simulink model "Test_Project_HLC"  (R2018a)
settings: Solver=FixedStepDiscrete  StartTime=0.0  StopTime=inf  FixedStep=1  RelTol=1e-3
undefined symbols (not defined in the file or in its folder): HLC
libraries: simulink x72, powerlib_meascontrol x1
settings Model: DataDictionary=HLC_DD.sldd  Creator=VIJAY BANDEPPA MURGE  LastModifiedBy=VIJAY BANDEPPA MURGE
settings DataIOCC: ReturnWorkspaceOutputs=on
settings SFSimCC: SimUseLocalCustomCode=on
settings RTWCC: RTWUseLocalCustomCode=on

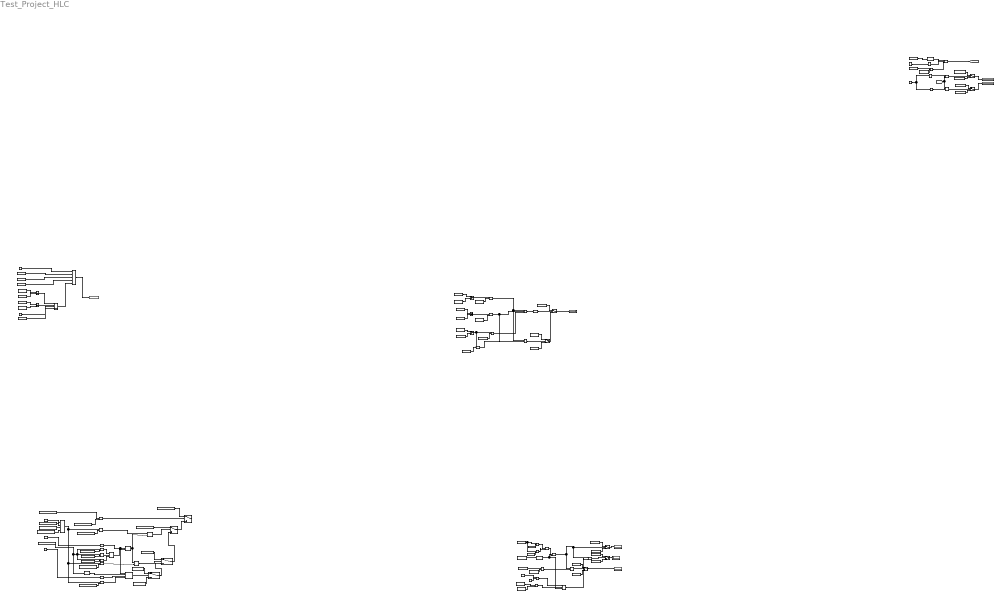
== system Test_Project_HLC ==
  note: Manual
  note: Vijay Murge
      | Road curvature
      | Wheel angle > 7° & Speed > 10km/h & High_Way/Express_Way/ Rural_Road/ Inside_City_Road/ Outside_City_Road
      | Curve_Adaptive_Right_Side_lamp
      |
      | Wheel angle > -7° & Speed > 10km/h & High_Way/Express_Way/ Rural_Road/ Inside_City_Road/ Outside_City_Road
      | Curve_Adaptive_Left_Side_lamp
  note: 4
      | Swapna Nerkar
      | Weather Conditions
      | Fog_Detected/Rain_detected & High_Way/Express_Way/ Rural_Road/Tunnel/Outside_City_Road
      | Fog_Lamp & Parking_Light
      |
      | Fog_Detected/Rain_detected & darkness & High_Way/ Express_Way/ Rural_Road/Tunnel/ Inside_City_Road/Outside_City_Road
      | Low Beam ,fog lamp and parking light
      |
      | Parked Vehicle
      | High_Way/Express_Way/ Rural_Road/Tunnel/Inside_City_Road/ Outside_City_Road & Ignition_On/Ignition_Off & Speed==0
      | Parking_Light
      |
      | Fog_Detected/Rain_detected/Inside_City_Road Fog lamp
  note: 3
      | Snehal Mane
      | Night-time running vehicle
      | Vehicle_Detected at 20m on Left_Side & Darkness & High_Way/Rural_Road/Outside_City_Road
      | Low_Beam -Left_Side_Headlamp
      |
      | Vehicle_Detected at 20m on Left_Side/Right _Side & Darkness & Inside_City_Road
      | Low_Beam
      |
      | Vehicle_Detected at 20m on Right_Side & Darkness & High_Way/Rural_Road/Inside_City_Road/Outside_City_Road
      | Low_Beam -Right_Side_Headlamp
      |
      | Speed > 60km/h & Darkness & No_Vehical_Detected & Inside_City_Road
      | High_Beam
  note: 1
      | Vikrant Gophane
      | Day-time running vehicle
      | Ignition_On/Ignition_Off & Day_Time
      | Headlight_Off
      |
      | Speed > 60km/h & Darkness & High_Way/Express_Way/ Rural_Road/Tunnel/Outside_City_Road
      | High_beam
      |
      | Ignition_On & Day_Time & InSide_City_Road
      | Low_Beam
  note: 2
      | Anupriya Gathekar
      | Day/Night Time but vehicle is in off mode
      | Darkness & Ignition_Off & Vehicle_Locked
      | Low_Beam for 15 Sec.
      |
      | Darkness & Ignition_Off & Vehicle_Unlocked
      | Low_Beam
  note: Auto_Mode
  AND{1,4..5,7..8,12..13} (7 alike) : Logic  IconShape=distinctive  AllPortsSameDT=off  OutDataTypeStr=boolean
  AND10 : Logic  Operator=OR  IconShape=distinctive  AllPortsSameDT=off  OutDataTypeStr=boolean
  AND{2..3,9,11} (4 alike) : Logic  Inputs=3  IconShape=distinctive  AllPortsSameDT=off  OutDataTypeStr=boolean
  AND6 : Logic  Inputs=4  IconShape=distinctive  AllPortsSameDT=off  OutDataTypeStr=boolean
  Angle : Constant  Value=-8
  Compare To Constant1 : simulink/Logic and Bit Operations/Compare To Constant  relop=>=  const=20  OutDataTypeStr=boolean
  Compare To Constant2 : simulink/Logic and Bit Operations/Compare To Constant  relop=>=  const=60  OutDataTypeStr=boolean
  Compare To Constant3 : simulink/Logic and Bit Operations/Compare To Constant  relop=>=  const=7  OutDataTypeStr=boolean
  Compare To Constant4 : simulink/Logic and Bit Operations/Compare To Constant  relop=>=  const=10  OutDataTypeStr=boolean
  Compare To Constant5 : simulink/Logic and Bit Operations/Compare To Constant  relop=<=  const=-7  OutDataTypeStr=boolean
  Constant2 : Constant
  Constant3 : Constant  Value=2
  Constant4 : Constant  Value=0
  Constant5 : Constant  Value=5
  Data Type Conversion : DataTypeConversion
  Data Type Conversion1 : DataTypeConversion
  Data Type Conversion2 : DataTypeConversion  OutDataTypeStr=boolean
  Detection_Distancet : Constant  Value=21
  Display{,1,3..7} (7 alike) : Display
  Enumerated Constant{,15..16,52,54} (5 alike) : simulink/Sources/Enumerated Constant  OutDataTypeStr=Enum: HLC  Value=HLC.Ignition_On  SampleTime=inf
  Enumerated Constant{1,6,17,41} (4 alike) : simulink/Sources/Enumerated Constant  OutDataTypeStr=Enum: HLC  Value=HLC.Day_Time  SampleTime=inf
  Enumerated Constant10 : simulink/Sources/Enumerated Constant  OutDataTypeStr=Enum: HLC  Value=HLC.Ignition_Off  SampleTime=inf
  Enumerated Constant11 : simulink/Sources/Enumerated Constant  OutDataTypeStr=Enum: HLC  Value=HLC.Ignition_Off  SampleTime=inf
  Enumerated Constant12 : simulink/Sources/Enumerated Constant  OutDataTypeStr=Enum: HLC  Value=HLC.Vehicle_locked  SampleTime=inf
  Enumerated Constant13 : simulink/Sources/Enumerated Constant  OutDataTypeStr=Enum: HLC  Value=HLC.Vehicle_Unlocked  SampleTime=inf
  Enumerated Constant{2,4..5,18..19,24,42} (7 alike) : simulink/Sources/Enumerated Constant  OutDataTypeStr=Enum: HLC  Value=HLC.Darkness  SampleTime=inf
  Enumerated Constant20 : simulink/Sources/Enumerated Constant  OutDataTypeStr=Enum: HLC  Value=HLC.Vehicle_locked  SampleTime=inf
  Enumerated Constant{21..22,39,43,65} (5 alike) : simulink/Sources/Enumerated Constant  OutDataTypeStr=Enum: HLC  Value=HLC.Low_Beam  SampleTime=inf
  Enumerated Constant23 : simulink/Sources/Enumerated Constant  OutDataTypeStr=Enum: HLC  Value=HLC.Vehicle_Unlocked  SampleTime=inf
  Enumerated Constant25 : simulink/Sources/Enumerated Constant  OutDataTypeStr=Enum: HLC  Value=HLC.High_Way  SampleTime=inf
  Enumerated Constant26 : simulink/Sources/Enumerated Constant  OutDataTypeStr=Enum: HLC  Value=HLC.Vehicle_Detected_Left  SampleTime=inf
  Enumerated Constant27 : simulink/Sources/Enumerated Constant  OutDataTypeStr=Enum: HLC  Value=HLC.Vehicle_Detected_Right  SampleTime=inf
  Enumerated Constant28 : simulink/Sources/Enumerated Constant  OutDataTypeStr=Enum: HLC  Value=HLC.Rural_Road  SampleTime=inf
  Enumerated Constant29 : simulink/Sources/Enumerated Constant  OutDataTypeStr=Enum: HLC  Value=HLC.Low_Beam_LHS  SampleTime=inf
  Enumerated Constant3 : simulink/Sources/Enumerated Constant  OutDataTypeStr=Enum: HLC  Value=HLC.Ignition_Off  SampleTime=inf
  Enumerated Constant30 : simulink/Sources/Enumerated Constant  OutDataTypeStr=Enum: HLC  Value=HLC.Outside_City_Road  SampleTime=inf
  Enumerated Constant31 : simulink/Sources/Enumerated Constant  OutDataTypeStr=Enum: HLC  Value=HLC.Vehicle_Detected_Left  SampleTime=inf
  Enumerated Constant32 : simulink/Sources/Enumerated Constant  OutDataTypeStr=Enum: HLC  Value=HLC.High_Way  SampleTime=inf
  Enumerated Constant33 : simulink/Sources/Enumerated Constant  OutDataTypeStr=Enum: HLC  Value=HLC.Vehicle_Detected_Right  SampleTime=inf
  Enumerated Constant34 : simulink/Sources/Enumerated Constant  OutDataTypeStr=Enum: HLC  Value=HLC.Low_Beam_RHS  SampleTime=inf
  Enumerated Constant35 : simulink/Sources/Enumerated Constant  OutDataTypeStr=Enum: HLC  Value=HLC.High_beam  SampleTime=inf
  Enumerated Constant37 : simulink/Sources/Enumerated Constant  OutDataTypeStr=Enum: HLC  Value=HLC.No_Vehical_Detected  SampleTime=inf
  Enumerated Constant38 : simulink/Sources/Enumerated Constant  OutDataTypeStr=Enum: HLC  Value=HLC.High_Way  SampleTime=inf
  Enumerated Constant40 : simulink/Sources/Enumerated Constant  OutDataTypeStr=Enum: HLC  Value=HLC.No_Vehical_Detected  SampleTime=inf
  Enumerated Constant{7,9,44,63} (4 alike) : simulink/Sources/Enumerated Constant  OutDataTypeStr=Enum: HLC  Value=HLC.Headlight_Off  SampleTime=inf
  Enumerated Constant45 : simulink/Sources/Enumerated Constant  OutDataTypeStr=Enum: HLC  Value=HLC.Fog_Detected  SampleTime=inf
  Enumerated Constant46 : simulink/Sources/Enumerated Constant  OutDataTypeStr=Enum: HLC  Value=HLC.Rain_Detected  SampleTime=inf
  Enumerated Constant47 : simulink/Sources/Enumerated Constant  OutDataTypeStr=Enum: HLC  Value=HLC.Inside_City_Road  SampleTime=inf
  Enumerated Constant48 : simulink/Sources/Enumerated Constant  OutDataTypeStr=Enum: HLC  Value=HLC.Fog_Lamp_ON  SampleTime=inf
  Enumerated Constant49 : simulink/Sources/Enumerated Constant  OutDataTypeStr=Enum: HLC  Value=HLC.Fog_Lamp_off  SampleTime=inf
  Enumerated Constant50 : simulink/Sources/Enumerated Constant  OutDataTypeStr=Enum: HLC  Value=HLC.Parking_Light_On  SampleTime=inf
  Enumerated Constant51 : simulink/Sources/Enumerated Constant  OutDataTypeStr=Enum: HLC  Value=HLC.Parking_Light_Off  SampleTime=inf
  Enumerated Constant53 : simulink/Sources/Enumerated Constant  OutDataTypeStr=Enum: HLC  Value=HLC.R_Ambient_Light_off  SampleTime=inf
  Enumerated Constant55 : simulink/Sources/Enumerated Constant  OutDataTypeStr=Enum: HLC  Value=HLC.L_Ambient_Light_On  SampleTime=inf
  Enumerated Constant56 : simulink/Sources/Enumerated Constant  OutDataTypeStr=Enum: HLC  Value=HLC.L_Ambient_Light_off  SampleTime=inf
  Enumerated Constant58 : simulink/Sources/Enumerated Constant  OutDataTypeStr=Enum: HLC  Value=HLC.R_Ambient_Light_On  SampleTime=inf
  Enumerated Constant64 : simulink/Sources/Enumerated Constant  OutDataTypeStr=Enum: HLC  Value=HLC.High_beam  SampleTime=inf
  Manual Switch : ManualSwitch  CurrentSetting=0
  Manual Switch1 : ManualSwitch
  Manual Switch2 : ManualSwitch  CurrentSetting=0
  Manual Switch3 : ManualSwitch  CurrentSetting=0
  Manual Switch4 : ManualSwitch
  Multiport Switch : MultiPortSwitch
  Multiport Switch1 : MultiPortSwitch  Inputs=4
  OR1 : Logic  Operator=OR  Inputs=3  IconShape=distinctive  AllPortsSameDT=off  OutDataTypeStr=boolean
  OR2 : Logic  Operator=OR  IconShape=distinctive  AllPortsSameDT=off  OutDataTypeStr=boolean
  On Dealy : powerlib_meascontrol/Logic/On Delay  DelayType=On delay  delay=4  ic=0  Ts=0
  Relational Operator{,1,3..7,9..16,18} (16 alike) : RelationalOperator  Operator===  OutDataTypeStr=boolean  RndMeth=Simplest
  Relational Operator17 : RelationalOperator  Operator=<=  OutDataTypeStr=boolean  RndMeth=Simplest
  Road_Types : simulink/Sources/Enumerated Constant  OutDataTypeStr=Enum: HLC  Value=HLC.Inside_City_Road  SampleTime=inf
  Speed : Constant  Value=70
  Speed_Check : Constant  Value=65
  Subsystem : Subsystem
  Switch{1..11} (11 alike) : Switch  Criteria=u2 > Threshold
  speed : Constant  Value=15
  wires:
  Enumerated Constant20/1 -> Relational Operator5/2
  AND2/1 -> On Dealy/1
  Manual Switch4/1 -> Relational Operator5/1, Relational Operator7/1
  Switch2/1 -> Display1/1
  Enumerated Constant18/1 -> Manual Switch2/2
  Enumerated Constant11/1 -> Relational Operator4/2
  Relational Operator3/1 -> AND3/1, AND2/1
  Enumerated Constant19/1 -> Relational Operator3/2
  Enumerated Constant10/1 -> Manual Switch3/2
  Enumerated Constant16/1 -> Manual Switch3/1
  Enumerated Constant12/1 -> Manual Switch4/1
  Enumerated Constant9/1 -> Switch2/1
  Manual Switch2/1 -> Relational Operator3/1
  Relational Operator5/1 -> AND2/3
  On Dealy/1 -> Switch2/2
  Enumerated Constant17/1 -> Manual Switch2/1
  Relational Operator4/1 -> AND3/2, AND2/2
  Manual Switch3/1 -> Relational Operator4/1
  Enumerated Constant13/1 -> Manual Switch4/2
  AND3/1 -> Switch3/2
  Enumerated Constant21/1 -> Switch3/1
  Enumerated Constant22/1 -> Switch3/3
  Enumerated Constant23/1 -> Relational Operator7/2
  Relational Operator7/1 -> AND3/3
  Switch3/1 -> Switch2/3
  Enumerated Constant26/1 -> Relational Operator6/2
  Enumerated Constant29/1 -> Switch4/1
  Switch4/1 -> Switch1/3
  Multiport Switch/1 -> Relational Operator12/1, Relational Operator13/1, Relational Operator6/1  "Vehiclae_Detection"
  Enumerated Constant33/1 -> Relational Operator12/2
  AND4/1 -> Switch5/2
  Enumerated Constant34/1 -> Switch5/1
  Switch5/1 -> Switch4/3
  AND1/1 -> AND5/2, AND4/1
  Relational Operator6/1 -> AND5/1
  AND5/1 -> Switch4/2
  Relational Operator12/1 -> AND4/2
  Detection_Distancet/1 -> Compare To Constant1/1  "Distance"
  Enumerated Constant28/1 -> Relational Operator10/2
  Relational Operator11/1 -> OR1/3
  Relational Operator10/1 -> OR1/2
  Enumerated Constant30/1 -> Relational Operator11/2
  Enumerated Constant32/1 -> Relational Operator9/2
  Relational Operator9/1 -> OR1/1
  Speed_Check/1 -> Compare To Constant2/1  "Speed"
  Enumerated Constant37/1 -> Relational Operator13/2
  Relational Operator13/1 -> AND6/4
  Compare To Constant2/1 -> AND6/3
  Enumerated Constant25/1 -> Data Type Conversion/1, Relational Operator11/1, Relational Operator10/1, Relational Operator9/1  "Road_Condition"
  Enumerated Constant35/1 -> Switch6/1
  Enumerated Constant39/1 -> Switch6/3
  Enumerated Constant31/1 -> Multiport Switch/3
  Enumerated Constant40/1 -> Multiport Switch/4
  Enumerated Constant27/1 -> Multiport Switch/2
  Constant2/1 -> Multiport Switch/1
  Data Type Conversion/1 -> AND6/2
  Enumerated Constant38/1 -> Data Type Conversion1/1
  Enumerated Constant15/1 -> Relational Operator16/1, Relational Operator15/1
  Enumerated Constant45/1 -> Relational Operator15/2
  Enumerated Constant46/1 -> Relational Operator16/2
  Relational Operator15/1 -> OR2/1
  Relational Operator16/1 -> OR2/2
  OR2/1 -> AND7/1
  AND7/1 -> Switch8/2, AND10/1, AND8/1
  Enumerated Constant41/1 -> Relational Operator14/1
  Relational Operator14/1 -> AND8/2
  Enumerated Constant42/1 -> Relational Operator14/2
  AND8/1 -> Switch7/2
  Enumerated Constant43/1 -> Switch7/1
  Enumerated Constant44/1 -> Switch7/3
  Switch7/1 -> Display5/1
  Constant5/1 -> Relational Operator17/2
  Constant4/1 -> Relational Operator17/1
  Relational Operator17/1 -> AND9/1
  Enumerated Constant52/1 -> Relational Operator18/1
  Relational Operator18/1 -> AND9/2
  Enumerated Constant54/1 -> Relational Operator18/2
  Data Type Conversion1/1 -> AND9/3, AND7/2
  AND10/1 -> Switch10/2
  Enumerated Constant48/1 -> Switch8/1
  Enumerated Constant49/1 -> Switch8/3
  Enumerated Constant50/1 -> Switch10/1
  Enumerated Constant51/1 -> Switch10/3
  AND9/1 -> AND10/2
  Switch10/1 -> Display3/1
  Switch8/1 -> Display4/1
  Enumerated Constant65/1 -> Multiport Switch1/4
  Enumerated Constant64/1 -> Multiport Switch1/3
  Enumerated Constant63/1 -> Multiport Switch1/2
  Constant3/1 -> Multiport Switch1/1
  Multiport Switch1/1 -> Display/1
  Enumerated Constant/1 -> Manual Switch/1
  Enumerated Constant3/1 -> Manual Switch/2
  Enumerated Constant4/1 -> Manual Switch1/2
  Enumerated Constant1/1 -> Manual Switch1/1
  Manual Switch/1 -> Subsystem/1(In1)
  Manual Switch1/1 -> Subsystem/2(In2)
  Speed/1 -> Subsystem/3(u)
  Road_Types/1 -> Subsystem/4(In4)
  Subsystem/1(Out1) -> Multiport Switch1/5
  Switch9/1 -> Display6/1
  Switch11/1 -> Display7/1
  Angle/1 -> Compare To Constant5/1, Compare To Constant3/1
  Compare To Constant4/1 -> AND11/2
  Compare To Constant5/1 -> AND13/2
  AND12/1 -> Switch9/2
  Compare To Constant3/1 -> AND12/1
  AND13/1 -> Switch11/2
  Data Type Conversion2/1 -> AND11/1
  AND11/1 -> [Road_Speed]
  [Road_Speed] -> AND12/2, AND13/1
  Enumerated Constant47/1 -> Data Type Conversion2/1
  speed/1 -> Compare To Constant4/1
  Enumerated Constant53/1 -> Switch9/3
  Enumerated Constant58/1 -> Switch9/1
  Enumerated Constant55/1 -> Switch11/1
  Enumerated Constant56/1 -> Switch11/3
  Enumerated Constant2/1 -> Relational Operator/1
  Relational Operator/1 -> AND11/3
  Enumerated Constant5/1 -> Relational Operator/2
  Compare To Constant1/1 -> AND6/1, AND1/1
  OR1/1 -> AND1/2
  Enumerated Constant24/1 -> Relational Operator1/1  "Night_day_check"
  Enumerated Constant6/1 -> Relational Operator1/2  "Night_day_check"
  Relational Operator1/1 -> Switch1/2
  Enumerated Constant7/1 -> Switch1/1
  ? -> ?
  Switch6/1 -> Switch5/3
  AND6/1 -> Switch6/2

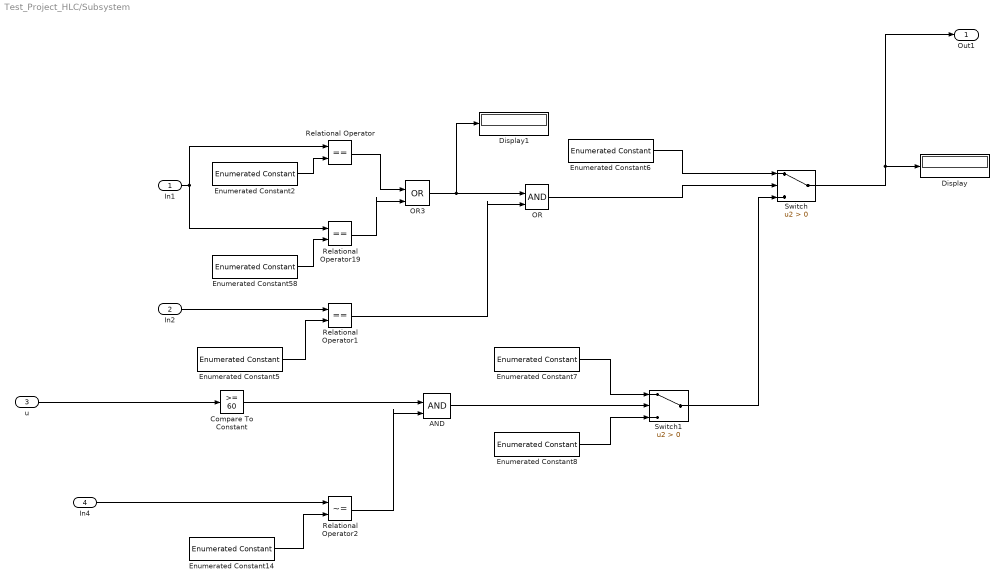
== system Test_Project_HLC/Subsystem ==
  In1 : Inport
  In2 : Inport  Port=2
  u : Inport  Port=3
  In4 : Inport  Port=4
  AND : Logic  IconShape=distinctive  AllPortsSameDT=off  OutDataTypeStr=boolean
  Compare To Constant : simulink/Logic and Bit Operations/Compare To Constant  relop=>=  const=60  OutDataTypeStr=boolean
  Display : Display
  Display1 : Display
  Enumerated Constant14 : simulink/Sources/Enumerated Constant  OutDataTypeStr=Enum: HLC  Value=HLC.Inside_City_Road  SampleTime=inf
  Enumerated Constant2 : simulink/Sources/Enumerated Constant  OutDataTypeStr=Enum: HLC  Value=HLC.Ignition_On  SampleTime=inf
  Enumerated Constant5 : simulink/Sources/Enumerated Constant  OutDataTypeStr=Enum: HLC  Value=HLC.Day_Time  SampleTime=inf
  Enumerated Constant58 : simulink/Sources/Enumerated Constant  OutDataTypeStr=Enum: HLC  Value=HLC.Ignition_Off  SampleTime=inf
  Enumerated Constant6 : simulink/Sources/Enumerated Constant  OutDataTypeStr=Enum: HLC  Value=HLC.Headlight_Off  SampleTime=inf
  Enumerated Constant7 : simulink/Sources/Enumerated Constant  OutDataTypeStr=Enum: HLC  Value=HLC.High_beam  SampleTime=inf
  Enumerated Constant8 : simulink/Sources/Enumerated Constant  OutDataTypeStr=Enum: HLC  Value=HLC.Low_Beam  SampleTime=inf
  OR : Logic  IconShape=distinctive  AllPortsSameDT=off  OutDataTypeStr=boolean
  OR3 : Logic  Operator=OR  IconShape=distinctive  AllPortsSameDT=off  OutDataTypeStr=boolean
  Relational Operator : RelationalOperator  Operator===  OutDataTypeStr=boolean  RndMeth=Simplest
  Relational Operator1 : RelationalOperator  Operator===  OutDataTypeStr=boolean  RndMeth=Simplest
  Relational Operator19 : RelationalOperator  Operator===  OutDataTypeStr=boolean  RndMeth=Simplest
  Relational Operator2 : RelationalOperator  Operator=~=  OutDataTypeStr=boolean  RndMeth=Simplest
  Switch : Switch  Criteria=u2 > Threshold
  Switch1 : Switch  Criteria=u2 > Threshold
  Out1 : Outport
  wires:
  Enumerated Constant5/1 -> Relational Operator1/2
  Relational Operator2/1 -> AND/2
  OR3/1 -> Display1/1, OR/1
  In4/1 -> Relational Operator2/1
  AND/1 -> Switch1/2
  OR/1 -> Switch/2
  Enumerated Constant6/1 -> Switch/1
  Enumerated Constant7/1 -> Switch1/1
  In1/1 -> Relational Operator19/1, Relational Operator/1
  Enumerated Constant2/1 -> Relational Operator/2
  Enumerated Constant14/1 -> Relational Operator2/2
  Relational Operator19/1 -> OR3/2
  Compare To Constant/1 -> AND/1
  Switch1/1 -> Switch/3
  Enumerated Constant8/1 -> Switch1/3
  Enumerated Constant58/1 -> Relational Operator19/2
  Relational Operator1/1 -> OR/2
  Relational Operator/1 -> OR3/1
  u/1 -> Compare To Constant/1
  In2/1 -> Relational Operator1/1
  Switch/1 -> Display/1, Out1/1
